simulink model "practica14simta"  (R2015a)
settings: Solver=ode45  StartTime=0.0  StopTime=10.0  RelTol=1e-3
settings Model: Creator=Alumnos  LastModifiedBy=Sala8

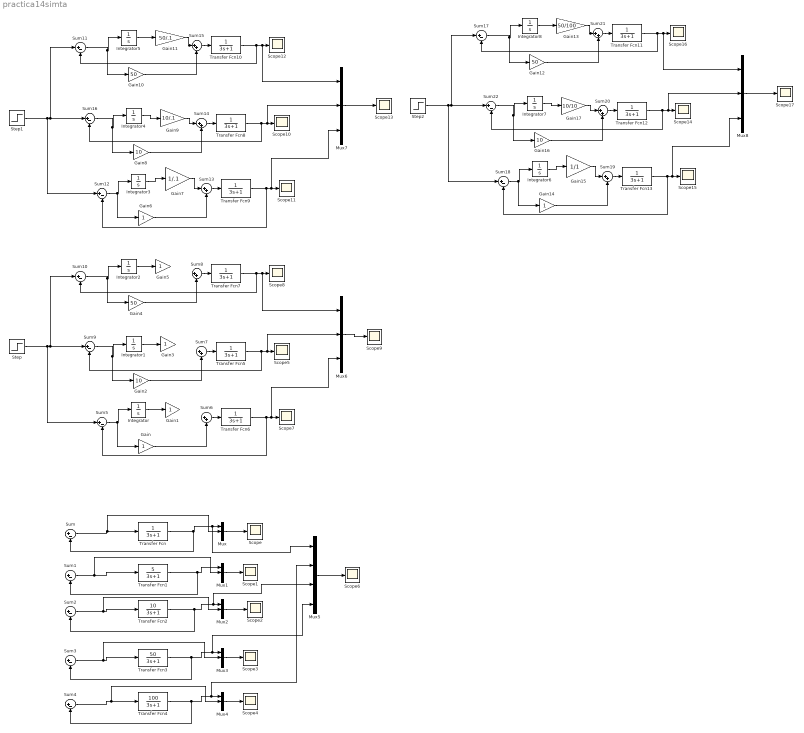
== system practica14simta ==
  Gain{,1,3,5..6,14} (6 alike) : Gain
  Gain10 : Gain  Gain=50
  Gain11 : Gain  Gain=50/.1
  Gain12 : Gain  Gain=50
  Gain13 : Gain  Gain=50/100
  Gain15 : Gain  Gain=1/1
  Gain16 : Gain  Gain=10
  Gain17 : Gain  Gain=10/10
  Gain2 : Gain  Gain=10
  Gain4 : Gain  Gain=50
  Gain7 : Gain  Gain=1/.1
  Gain8 : Gain  Gain=10
  Gain9 : Gain  Gain=10/.1
  Integrator{,1..8} (9 alike) : Integrator
  Mux{,1..4,6..8} (8 alike) : Mux  Inputs=3
  Mux5 : Mux
  Scope{,1..17} (18 alike) : Scope
      Scope10 settings: SaveName=ScopeData10
      Scope11 settings: SaveName=ScopeData11
      Scope12 settings: SaveName=ScopeData12
      Scope13 settings: SaveName=ScopeData13
      Scope14 settings: SaveName=ScopeData14
      Scope15 settings: SaveName=ScopeData15
      Scope16 settings: SaveName=ScopeData16
      Scope17 settings: SaveName=ScopeData17
      Scope2 settings: SaveName=ScopeData2
      Scope3 settings: SaveName=ScopeData3
      Scope4 settings: SaveName=ScopeData4
      Scope5 settings: SaveName=ScopeData5
      Scope6 settings: SaveName=ScopeData6
      Scope7 settings: SaveName=ScopeData7
      Scope8 settings: SaveName=ScopeData8
      Scope9 settings: SaveName=ScopeData9
  Step : Step  SampleTime=0
  Step1 : Step  SampleTime=0
  Step2 : Step  SampleTime=0
  Sum{,1..5,9..12,16..18,22} (14 alike) : Sum  Inputs=|+-
  Sum{6..8,13..15,19..21} (9 alike) : Sum  Inputs=|++
  Transfer Fcn{,5..13} (10 alike) : TransferFcn  Denominator=[3 1]
  Transfer Fcn1 : TransferFcn  Numerator=[5]  Denominator=[3 1]
  Transfer Fcn2 : TransferFcn  Numerator=[10]  Denominator=[3 1]
  Transfer Fcn3 : TransferFcn  Numerator=[50]  Denominator=[3 1]
  Transfer Fcn4 : TransferFcn  Numerator=[100]  Denominator=[3 1]
  wires:
  Sum/1 -> Mux/2, Transfer Fcn/1
  Transfer Fcn/1 -> Sum/2, Mux5/1, Mux/1
  ? -> Sum/1, Sum1/1, Sum2/1, Sum3/1, Sum4/1, Mux4/3, Mux3/3, Mux2/3, Mux1/3, Mux/3
  Transfer Fcn1/1 -> Sum1/2, Mux1/1
  Sum1/1 -> Mux1/2, Transfer Fcn1/1
  Sum3/1 -> Mux3/2, Transfer Fcn3/1
  Sum2/1 -> Mux2/2, Transfer Fcn2/1
  Transfer Fcn2/1 -> Sum2/2, Mux5/3, Mux2/1
  Transfer Fcn3/1 -> Sum3/2, Mux5/4, Mux3/1
  Transfer Fcn4/1 -> Sum4/2, Mux5/2, Mux4/1
  Sum4/1 -> Mux4/2, Transfer Fcn4/1
  Mux2/1 -> Scope2/1
  Mux1/1 -> Scope1/1
  Mux/1 -> Scope/1
  Mux3/1 -> Scope3/1
  Mux4/1 -> Scope4/1
  Transfer Fcn6/1 -> Sum5/2, Mux6/3, Scope7/1
  Mux5/1 -> Scope6/1
  Sum5/1 -> Gain/1, Integrator/1
  Sum6/1 -> Transfer Fcn6/1
  Integrator/1 -> Gain1/1
  Gain/1 -> Sum6/2
  Transfer Fcn5/1 -> Sum9/2, Mux6/2, Scope5/1
  Sum9/1 -> Integrator1/1, Gain2/1
  Sum7/1 -> Transfer Fcn5/1
  Integrator1/1 -> Gain3/1
  Gain2/1 -> Sum7/2
  Transfer Fcn7/1 -> Sum10/2, Mux6/1, Scope8/1
  Sum10/1 -> Gain4/1, Integrator2/1
  Sum8/1 -> Transfer Fcn7/1
  Integrator2/1 -> Gain5/1
  Gain4/1 -> Sum8/2
  Step/1 -> Sum5/1, Sum9/1, Sum10/1
  Mux6/1 -> Scope9/1
  Transfer Fcn9/1 -> Scope11/1, Mux7/3, Sum12/2
  Sum12/1 -> Integrator3/1, Gain6/1
  Sum13/1 -> Transfer Fcn9/1
  Integrator3/1 -> Gain7/1
  Gain6/1 -> Sum13/2
  Transfer Fcn8/1 -> Scope10/1, Mux7/2, Sum16/2
  Sum16/1 -> Gain8/1, Integrator4/1
  Sum14/1 -> Transfer Fcn8/1
  Integrator4/1 -> Gain9/1
  Gain8/1 -> Sum14/2
  Transfer Fcn10/1 -> Scope12/1, Mux7/1, Sum11/2
  Sum11/1 -> Integrator5/1, Gain10/1
  Sum15/1 -> Transfer Fcn10/1
  Integrator5/1 -> Gain11/1
  Gain10/1 -> Sum15/2
  Step1/1 -> Sum11/1, Sum16/1, Sum12/1
  Mux7/1 -> Scope13/1
  Gain7/1 -> Sum13/1
  Gain9/1 -> Sum14/1
  Gain11/1 -> Sum15/1
  Transfer Fcn13/1 -> Sum18/2, Mux8/3, Scope15/1
  Sum18/1 -> Gain14/1, Integrator6/1
  Sum19/1 -> Transfer Fcn13/1
  Integrator6/1 -> Gain15/1
  Gain14/1 -> Sum19/2
  Transfer Fcn12/1 -> Sum22/2, Mux8/2, Scope14/1
  Sum22/1 -> Integrator7/1, Gain16/1
  Sum20/1 -> Transfer Fcn12/1
  Integrator7/1 -> Gain17/1
  Gain16/1 -> Sum20/2
  Transfer Fcn11/1 -> Sum17/2, Mux8/1, Scope16/1
  Sum17/1 -> Gain12/1, Integrator8/1
  Sum21/1 -> Transfer Fcn11/1
  Integrator8/1 -> Gain13/1
  Gain12/1 -> Sum21/2
  Step2/1 -> Sum18/1, Sum22/1, Sum17/1
  Mux8/1 -> Scope17/1
  Gain15/1 -> Sum19/1
  Gain17/1 -> Sum20/1
  Gain13/1 -> Sum21/1
